simulink library "VariableOrderDifferentialEquationsToolbox"  (R2020a)
settings: Solver=VariableStepAuto  StartTime=0.0  StopTime=10.0  RelTol=1e-3
(part 1 of 3)
settings Model: Creator=dell-wi  LastModifiedBy=Pio
settings DataIOCC: ReturnWorkspaceOutputs=off
settings DebuggingCC: ArithmeticOperatorsInVariantConditions=warning
settings SFSimCC: SimUseLocalCustomCode=off  CustomCodeUndefinedFunction=UseInterfaceOnly
settings RTWCC: RTWUseLocalCustomCode=off

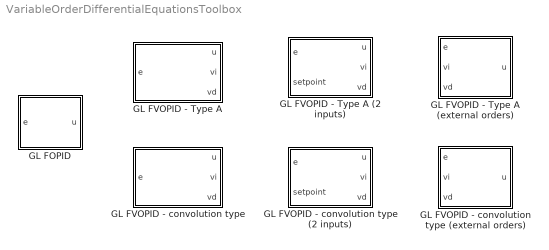
== system VariableOrderDifferentialEquationsToolbox ==
  GL FOPID : Subsystem  mask{kp=1, ki=1, kd=0, sampleTime=1, inputBufferSize=-1, constantIntegralOrder=1, constantDerivativeOrder=1, satEnab=off, satHigh=inf, satLow=-inf}
      mask prompts: kp "Proportional (P)"; ki "Integral (I)"; kd "Derivative (D)"; sampleTime "Sample time"; inputBufferSize "Input buffer size (-1 for automatically calculated)"; constantIntegralOrder "Integral order"; constantDerivativeOrder "Derivative order"; satEnab "Limit output"; satHigh "Upper limit"; satLow "Lower limit"
      mask init:
      | % Initialize block parameters
      | fvopidToolbox.library.utils.initializeBasicModelParameters(sampleTime, inputBufferSize,'fopid');
      settings: CopyFcn=set_param(gcbh, 'LinkStatus', 'none');
      mask Callback satEnab:
      | limitOutputCheckBoxValue = get_param(gcb,'satEnab');
      | if strcmp(limitOutputCheckBoxValue, 'on')
      |    fvopidToolbox.library.utils.setMaskParameterPropertyValue('satHigh', 'MaskEnables', 'on');
      |    fvopidToolbox.library.utils.setMaskParameterPropertyValue('satLow', 'MaskEnables', 'on');
      | else
      |    fvopidToolbox.library.utils.setMaskParameterPropertyValue('satHigh', 'MaskEnables', 'off');
      |    fvopidToolbox.library.utils.setMaskParameterPropertyValue('satLow', 'MaskEnables', 'off');
      | end
      mask DialogControl mainTab Prompt: Main
      mask DialogControl controllerParametersGroupBox Prompt: Controller parameters
      mask DialogControl outputSaturationTab Prompt: Output saturation
      mask DialogControl outputSaturationGroupBox Prompt: Output saturation
  GL FVOPID - Type A : Subsystem  mask{kp=1, ki=1, kd=0, sampleTime=1, inputBufferSize=-1, satEnab=off, satHigh=inf, satLow=-inf, integralOrderTypePopup=Constant order, constantIntegralOrder=1, integralErrorToSetpointRatio=off, integralErrorValuesVector=[0.2, 0.4, 0.6, 0.8], integralOrderValuesVector=[1, 2, 3, 4, 5], timeDependentIntegralOrderExpression=3 * t + 2 * e, derivativeOrderTypePopup=Constant order, constantDerivativeOrder=1, derivativeErrorToSetpointRatio=off, derivativeErrorValuesVector=[0.2, 0.4, 0.6, 0.8], derivativeOrderValuesVector=[1, 2, 3, 4, 5], timeDependentDerivativeOrderExpression=2*t + e}
      mask prompts: kp "Proportional (P)"; ki "Integral (I)"; kd "Derivative (D)"; sampleTime "Sample time"; inputBufferSize "Input buffer size (-1 for automatically calculated)"; satEnab "Limit output"; satHigh "Upper limit"; satLow "Lower limit"; integralOrderTypePopup "Integral order type"; constantIntegralOrder "Integral order"; integralErrorToSetpointRatio "Use error/setpoint ratio"; integralErrorValuesVector "Vector of control error values"; integralOrderValuesVector "Vector of order values"; derivativeOrderTypePopup "Derivative order type"; constantDerivativeOrder "Derivative order"; derivativeErrorToSetpointRatio "Use error/setpoint ratio"; derivativeErrorValuesVector "Vector of control error values"; derivativeOrderValuesVector "Vector of order values"
      mask init:
      | % Initialize block parameters
      | fvopidToolbox.library.utils.initializeBasicModelParameters(sampleTime, inputBufferSize,'fvopidOptimized');
      | integralOrderTypeComboBoxValue = get_param(gcb,'integralOrderTypePopup');
      | derivativeOrderTypeComboBoxValue = get_param(gcb,'derivativeOrderTypePopup');
      | 
      | % Set order function type
      | switch integralOrderTypeComboBoxValue
      |     case 'Constant order'
      |         integralOrderType = 1;
      |     case 'Function of control error'
      |         integralErrorToSetpointRatioValue = get_param(gcb,'integralErrorToSetpointRatio');
      |         if strcmp(integralErrorToSetpointRatioValue, 'on')
      |             integralOrderType = 3;
      |         else
      |             integralOrderType = 2;
      |         end
      |     otherwise
      |         integralOrderExpressionCode = get_param(gcb,'timeDependentIntegralOrderExpression');
      |         newScript = sprintf(['function y = integralTimeDependentMatlabFunction(t, e)\n'...
      |             'y = '  integralOrderExpressionCode ';\nend']);
      |         fvopidToolbox.utils.updateMatlabFunctionBlockScript('integralTimeDependentBlock', newScript,...
      |             [gcb '/integralTimeDependentSubsystem/integralTimeDependentBlock']);
      |         integralOrderType = 4;
      | end
      | 
      | switch derivativeOrderTypeComboBoxValue
      |     case 'Constant order'
      |         derivativeOrderType = 1;
      |     case 'Function of control error'
      |         derivatieErrorToSetpointRatioValue = get_param(gcb,'derivativeErrorToSetpointRatio');
      |         if strcmp(derivatieErrorToSetpointRatioValue, 'on')
      |             derivativeOrderType = 3;
      |         else
      |             derivativeOrderType = 2;
      |         end
      |     otherwise
      |         derivativeOrderExpressionCode = get_param(gcb,'timeDependentDerivativeOrderExpression');
      |         newScript = sprintf(['function y = derivativeTimeDependentMatlabFunction(t, e)\n'...
      |             'y = ' derivativeOrderExpressionCode ';\nend']);
      |         fvopidToolbox.utils.updateMatlabFunctionBlockScript('derivativeTimeDependentBlock', newScript,...
      |             [gcb '/derivativeTimeDependentSubsystem/derivativeTimeDependentBlock']);
      |         derivativeOrderType = 4;
      | end
      | 
      | % Update the input ports
      | setpointInputBlock = find_system(gcb,...
      |     'LookUnderMasks','on',...
      |     'FollowLinks','on','Name','setpointInput');
      | 
      | integralSetpointHolderBlock = find_system(gcb,...
      |     'LookUnderMasks','on',...
      |     'FollowLinks','on','Name','integral_setpoint_placeHolder');
      | 
      | derivativeSetpointHolderBlock = find_system(gcb,...
      |     'LookUnderMasks','on',...
      |     'FollowLinks','on','Name','derivative_setpoint_placeHolder');
      | 
      | if integralOrderType == 3 || derivativeOrderType == 3
      |     if isempty(setpointInputBlock)
      |         add_block('built-in/Inport',[gcb,'/setpointInput']);  
      |     else
      |         h = get_param([gcb '/setpointInput'], 'LineHandles'); 
      |         delete_line(h.Outport(1));
      |     end
      | 
      |     if integralOrderType == 3
      |         if ~isempty(integralSetpointHolderBlock)
      |             h = get_param([gcb '/integral_setpoint_placeHolder'], 'LineHandles'); 
      |             delete_line(h.Outport(1));
      |             delete_block(integralSetpointHolderBlock);
      |         end
      |         add_line(gcb,'setpointInput/1','integralRatioDependentSubsystem/2');
      |     else
      |         if isempty(integralSetpointHolderBlock)
      |             add_block('built-in/Constant',[gcb,'/integral_setpoint_placeHolder']);
      |             set_param([gcb '/integral_setpoint_placeHolder'], 'Value', '0');
      |             add_line(gcb,'integral_setpoint_placeHolder/1','integralRatioDependentSubsystem/2');
      |         end
      |     end
      | 
      |     if derivativeOrderType == 3
      |         if ~isempty(derivativeSetpointHolderBlock)
      |             h = get_param([gcb '/derivative_setpoint_placeHolder'], 'LineHandles'); 
      |             delete_line(h.Outport(1));
      |             delete_block(derivativeSetpointHolderBlock);
      |         end
      |         add_line(gcb,'setpointInput/1','derivativeRatioDependentSubsystem/2');
      |     else
      |         if isempty(derivativeSetpointHolderBlock)
      |             add_block('built-in/Constant',[gcb,'/derivative_setpoint_placeHolder']);
      |             set_param([gcb '/derivative_setpoint_placeHolder'], 'Value', '0');
      |             add_line(gcb,'derivative_setpoint_placeHolder/1','derivativeRatioDependentSubsystem/2');
      |         end
      |     end
      | else
      |     if ~isempty(setpointInputBlock)
      |         h = get_param([gcb '/setpointInput'], 'LineHandles'); 
      |         delete_line(h.Outport(1));
      |         delete_block(setpointInputBlock);
      |     end
      |     
      |     if isempty(integralSetpointHolderBlock)
      |         add_block('built-in/Constant',[gcb,'/integral_setpoint_placeHolder']);
      |         set_param([gcb '/integral_setpoint_placeHolder'], 'Value', '0');
      |         add_line(gcb,'integral_setpoint_placeHolder/1','integralRatioDependentSubsystem/2');
      |     end
      |     
      |     if isempty(derivativeSetpointHolderBlock)
      |         add_block('built-in/Constant',[gcb,'/derivative_setpoint_placeHolder']);
      |         set_param([gcb '/derivative_setpoint_placeHolder'], 'Value', '0');
      |         add_line(gcb,'derivative_setpoint_placeHolder/1','derivativeRatioDependentSubsystem/2');
      |     end
      | end
      settings: CopyFcn=set_param(gcbh, 'LinkStatus', 'none');
      mask Callback satEnab:
      | limitOutputCheckBoxValue = get_param(gcb,'satEnab');
      | if strcmp(limitOutputCheckBoxValue, 'on')
      |    fvopidToolbox.library.utils.setMaskParameterPropertyValue('satHigh', 'MaskEnables', 'on');
      |    fvopidToolbox.library.utils.setMaskParameterPropertyValue('satLow', 'MaskEnables', 'on');
      | else
      |    fvopidToolbox.library.utils.setMaskParameterPropertyValue('satHigh', 'MaskEnables', 'off');
      |    fvopidToolbox.library.utils.setMaskParameterPropertyValue('satLow', 'MaskEnables', 'off');
      | end
      mask TypeOptions integralOrderTypePopup: Constant order | Function of control error | User defined expression
      mask Callback integralOrderTypePopup:
      | selectedComboBoxValue = get_param(gcb,'integralOrderTypePopup');
      | 
      | switch selectedComboBoxValue
      |     case 'Constant order'
      |         fvopidToolbox.library.utils.setMaskElementVisiblePropertyValue('constantIntegralOrderPanel', 'on');
      |         fvopidToolbox.library.utils.setMaskElementVisiblePropertyValue('controlErrorDependentIntegralOrderPanel', 'off');
      |         fvopidToolbox.library.utils.setMaskElementVisiblePropertyValue('timeDependentIntegralOrderPanel', 'off');
      |     case 'Function of control error'
      |         fvopidToolbox.library.utils.setMaskElementVisiblePropertyValue('constantIntegralOrderPanel', 'off');
      |         fvopidToolbox.library.utils.setMaskElementVisiblePropertyValue('controlErrorDependentIntegralOrderPanel', 'on');
      |         fvopidToolbox.library.utils.setMaskElementVisiblePropertyValue('timeDependentIntegralOrderPanel', 'off');
      |     otherwise
      |         fvopidToolbox.library.utils.setMaskElementVisiblePropertyValue('constantIntegralOrderPanel', 'off');
      |         fvopidToolbox.library.utils.setMaskElementVisiblePropertyValue('controlErrorDependentIntegralOrderPanel', 'off');
      |         fvopidToolbox.library.utils.setMaskElementVisiblePropertyValue('timeDependentIntegralOrderPanel', 'on');
      | end
      mask TypeOptions derivativeOrderTypePopup: Constant order | Function of control error | User defined expression
      mask Callback derivativeOrderTypePopup:
      | selectedComboBoxValue = get_param(gcb,'derivativeOrderTypePopup');
      | 
      | switch selectedComboBoxValue
      |     case 'Constant order'
      |         fvopidToolbox.library.utils.setMaskElementVisiblePropertyValue('constantDerivativeOrderPanel', 'on');
      |         fvopidToolbox.library.utils.setMaskElementVisiblePropertyValue('controlErrorDependentDerivativeOrderPanel', 'off');
      |         fvopidToolbox.library.utils.setMaskElementVisiblePropertyValue('timeDependentDerivativeOrderPanel', 'off');
      |     case 'Function of control error'
      |         fvopidToolbox.library.utils.setMaskElementVisiblePropertyValue('constantDerivativeOrderPanel', 'off');
      |         fvopidToolbox.library.utils.setMaskElementVisiblePropertyValue('controlErrorDependentDerivativeOrderPanel', 'on');
      |         fvopidToolbox.library.utils.setMaskElementVisiblePropertyValue('timeDependentDerivativeOrderPanel', 'off');
      |     otherwise
      |         fvopidToolbox.library.utils.setMaskElementVisiblePropertyValue('constantDerivativeOrderPanel', 'off');
      |         fvopidToolbox.library.utils.setMaskElementVisiblePropertyValue('controlErrorDependentDerivativeOrderPanel', 'off');
      |         fvopidToolbox.library.utils.setMaskElementVisiblePropertyValue('timeDependentDerivativeOrderPanel', 'on');
      | end
      mask DialogControl mainTab Prompt: Main
      mask DialogControl controllerParametersGroupBox Prompt: Controller parameters
      mask DialogControl outputSaturationTab Prompt: Output saturation
      mask DialogControl outputSaturationGroupBox Prompt: Output saturation
      mask DialogControl integralOrderTab Prompt: Integral order
      mask DialogControl errorDependentIntegralOrderDescription1 Prompt: Provide a vector of control error values and a vector of order vales. Vector of order values should have one element more than the vector of error. E.g. for if the vector of error values is: [e1, e2, e3] and the vector of orders is [o1, o2, o3, o4], then the orders are generated according to the following rule:
      mask DialogControl errorDependentIntegralOrderDescription2 Prompt: - order = o1 for errors < e1,
      mask DialogControl errorDependentIntegralOrderDescription3 Prompt: - order = o2 for e1 <= error < e2,
      mask DialogControl errorDependentIntegralOrderDescription4 Prompt: - order = o3 for e2 <= error < e3,
      mask DialogControl errorDependentIntegralOrderDescription5 Prompt: - order = o4 for error >= e3.
      mask DialogControl timeDependentIntegralOrderDescription1 Prompt: Insert a short expression which returns value of order as a function of time (t) and/or control error (e), e.g.: '2*t + e' (where 't' is current simulation time and 'e' is current value of the control error).
      mask DialogControl derivativeOrderTab Prompt: Derivative order
      mask DialogControl errorDependentDerivativeOrderDescription1 Prompt: Provide a vector of control error values and a vector of order vales. Vector of order values should have one element more than the vector of error. E.g. for if the vector of order values is: [e1, e2, e3] and the vector of orders is [o1, o2, o3, o4], then the orders are generated according to the following rule:
      mask DialogControl errorDependentDerivativeOrderDescription2 Prompt: - order = o1 for errors > e1,
      mask DialogControl errorDependentDerivativeOrderDescription3 Prompt: - order = o2 for e2 < error <= e1,
      mask DialogControl errorDependentDerivativeOrderDescription4 Prompt: - order = o3 for e3 < error <= e2,
      mask DialogControl errorDependentDerivativeOrderDescription5 Prompt: - order = o4 for error < e3.
      mask DialogControl timeDependentDerivativeOrderDescription1 Prompt: Insert short expression which returns value of order as a function of time (t) and/or control error (e), e.g.: '2*t + e' (where 't' is current simulation time and 'e' is current value of the control error).
  GL FVOPID - Type A (2 inputs) : Subsystem  mask{kp=1, ki=1, kd=0, sampleTime=1, inputBufferSize=-1, satEnab=off, satHigh=inf, satLow=-inf, integralOrderTypePopup=Constant order, constantIntegralOrder=1, integralErrorToSetpointRatio=off, integralErrorValuesVector=[0.2, 0.4, 0.6, 0.8], integralOrderValuesVector=[1, 2, 3, 4, 5], timeDependentIntegralOrderExpression=3 * t + 2 * e, derivativeOrderTypePopup=Constant order, constantDerivativeOrder=1, derivativeErrorToSetpointRatio=off, derivativeErrorValuesVector=[0.2, 0.4, 0.6, 0.8], derivativeOrderValuesVector=[1, 2, 3, 4, 5], timeDependentDerivativeOrderExpression=2*t + e}
      mask prompts: kp "Proportional (P)"; ki "Integral (I)"; kd "Derivative (D)"; sampleTime "Sample time"; inputBufferSize "Input buffer size (-1 for automatically calculated)"; satEnab "Limit output"; satHigh "Upper limit"; satLow "Lower limit"; integralOrderTypePopup "Integral order type"; constantIntegralOrder "Integral order"; integralErrorToSetpointRatio "Use error/setpoint ratio"; integralErrorValuesVector "Vector of control error values"; integralOrderValuesVector "Vector of order values"; derivativeOrderTypePopup "Derivative order type"; constantDerivativeOrder "Derivative order"; derivativeErrorToSetpointRatio "Use error/setpoint ratio"; derivativeErrorValuesVector "Vector of control error values"; derivativeOrderValuesVector "Vector of order values"
      mask init:
      | % Initialize block parameters
      | fvopidToolbox.library.utils.initializeBasicModelParameters(sampleTime, inputBufferSize,'fvopidOptimized');
      | integralOrderTypeComboBoxValue = get_param(gcb,'integralOrderTypePopup');
      | derivativeOrderTypeComboBoxValue = get_param(gcb,'derivativeOrderTypePopup');
      | 
      | % Set order function type
      | switch integralOrderTypeComboBoxValue
      |     case 'Constant order'
      |         integralOrderType = 1;
      |     case 'Function of control error'
      |         integralErrorToSetpointRatioValue = get_param(gcb,'integralErrorToSetpointRatio');
      |         if strcmp(integralErrorToSetpointRatioValue, 'on')
      |             integralOrderType = 3;
      |         else
      |             integralOrderType = 2;
      |         end
      |     otherwise
      |         integralOrderExpressionCode = get_param(gcb,'timeDependentIntegralOrderExpression');
      |         newScript = sprintf(['function y = integralTimeDependentMatlabFunction(t, e)\n'...
      |             'y = '  integralOrderExpressionCode ';\nend']);
      |         fvopidToolbox.utils.updateMatlabFunctionBlockScript('integralTimeDependentBlock', newScript,...
      |             [gcb '/integralTimeDependentSubsystem/integralTimeDependentBlock']);
      |         integralOrderType = 4;
      | end
      | 
      | switch derivativeOrderTypeComboBoxValue
      |     case 'Constant order'
      |         derivativeOrderType = 1;
      |     case 'Function of control error'
      |         derivatieErrorToSetpointRatioValue = get_param(gcb,'derivativeErrorToSetpointRatio');
      |         if strcmp(derivatieErrorToSetpointRatioValue, 'on')
      |             derivativeOrderType = 3;
      |         else
      |             derivativeOrderType = 2;
      |         end
      |     otherwise
      |         derivativeOrderExpressionCode = get_param(gcb,'timeDependentDerivativeOrderExpression');
      |         newScript = sprintf(['function y = derivativeTimeDependentMatlabFunction(t, e)\n'...
      |             'y = ' derivativeOrderExpressionCode ';\nend']);
      |         fvopidToolbox.utils.updateMatlabFunctionBlockScript('derivativeTimeDependentBlock', newScript,...
      |             [gcb '/derivativeTimeDependentSubsystem/derivativeTimeDependentBlock']);
      |         derivativeOrderType = 4;
      | end
      | 
      | % Update the input ports
      | setpointInputBlock = find_system(gcb,...
      |     'LookUnderMasks','on',...
      |     'FollowLinks','on','Name','setpointInput');
      | if integralOrderType == 3 || derivativeOrderType == 3
      |     if isempty(setpointInputBlock)
      |         add_block('built-in/Inport',[gcb,'/setpointInput']);  
      |     else
      |         h = get_param([gcb '/setpointInput'], 'LineHandles'); 
      |         delete_line(h.Outport(1));
      |     end
      | 
      |     if integralOrderType == 3
      |         add_line(gcb,'setpointInput/1','integralRatioDependentSubsystem/2');
      |     end
      | 
      |     if derivativeOrderType == 3
      |         add_line(gcb,'setpointInput/1','derivativeRatioDependentSubsystem/2');
      |     end
      | else
      |     if ~isempty(setpointInputBlock)
      |         h = get_param([gcb '/setpointInput'], 'LineHandles'); 
      |         delete_line(h.Outport(1));
      |         delete_block(setpointInputBlock);
      |     end
      | end
      settings: CopyFcn=set_param(gcbh, 'LinkStatus', 'none');
      mask Callback satEnab:
      | limitOutputCheckBoxValue = get_param(gcb,'satEnab');
      | if strcmp(limitOutputCheckBoxValue, 'on')
      |    fvopidToolbox.library.utils.setMaskParameterPropertyValue('satHigh', 'MaskEnables', 'on');
      |    fvopidToolbox.library.utils.setMaskParameterPropertyValue('satLow', 'MaskEnables', 'on');
      | else
      |    fvopidToolbox.library.utils.setMaskParameterPropertyValue('satHigh', 'MaskEnables', 'off');
      |    fvopidToolbox.library.utils.setMaskParameterPropertyValue('satLow', 'MaskEnables', 'off');
      | end
      mask TypeOptions integralOrderTypePopup: Constant order | Function of control error | User defined expression
      mask Callback integralOrderTypePopup:
      | selectedComboBoxValue = get_param(gcb,'integralOrderTypePopup');
      | 
      | switch selectedComboBoxValue
      |     case 'Constant order'
      |         fvopidToolbox.library.utils.setMaskElementVisiblePropertyValue('constantIntegralOrderPanel', 'on');
      |         fvopidToolbox.library.utils.setMaskElementVisiblePropertyValue('controlErrorDependentIntegralOrderPanel', 'off');
      |         fvopidToolbox.library.utils.setMaskElementVisiblePropertyValue('timeDependentIntegralOrderPanel', 'off');
      |     case 'Function of control error'
      |         fvopidToolbox.library.utils.setMaskElementVisiblePropertyValue('constantIntegralOrderPanel', 'off');
      |         fvopidToolbox.library.utils.setMaskElementVisiblePropertyValue('controlErrorDependentIntegralOrderPanel', 'on');
      |         fvopidToolbox.library.utils.setMaskElementVisiblePropertyValue('timeDependentIntegralOrderPanel', 'off');
      |     otherwise
      |         fvopidToolbox.library.utils.setMaskElementVisiblePropertyValue('constantIntegralOrderPanel', 'off');
      |         fvopidToolbox.library.utils.setMaskElementVisiblePropertyValue('controlErrorDependentIntegralOrderPanel', 'off');
      |         fvopidToolbox.library.utils.setMaskElementVisiblePropertyValue('timeDependentIntegralOrderPanel', 'on');
      | end
      mask TypeOptions derivativeOrderTypePopup: Constant order | Function of control error | User defined expression
      mask Callback derivativeOrderTypePopup:
      | selectedComboBoxValue = get_param(gcb,'derivativeOrderTypePopup');
      | 
      | switch selectedComboBoxValue
      |     case 'Constant order'
      |         fvopidToolbox.library.utils.setMaskElementVisiblePropertyValue('constantDerivativeOrderPanel', 'on');
      |         fvopidToolbox.library.utils.setMaskElementVisiblePropertyValue('controlErrorDependentDerivativeOrderPanel', 'off');
      |         fvopidToolbox.library.utils.setMaskElementVisiblePropertyValue('timeDependentDerivativeOrderPanel', 'off');
      |     case 'Function of control error'
      |         fvopidToolbox.library.utils.setMaskElementVisiblePropertyValue('constantDerivativeOrderPanel', 'off');
      |         fvopidToolbox.library.utils.setMaskElementVisiblePropertyValue('controlErrorDependentDerivativeOrderPanel', 'on');
      |         fvopidToolbox.library.utils.setMaskElementVisiblePropertyValue('timeDependentDerivativeOrderPanel', 'off');
      |     otherwise
      |         fvopidToolbox.library.utils.setMaskElementVisiblePropertyValue('constantDerivativeOrderPanel', 'off');
      |         fvopidToolbox.library.utils.setMaskElementVisiblePropertyValue('controlErrorDependentDerivativeOrderPanel', 'off');
      |         fvopidToolbox.library.utils.setMaskElementVisiblePropertyValue('timeDependentDerivativeOrderPanel', 'on');
      | end
      mask DialogControl mainTab Prompt: Main
      mask DialogControl controllerParametersGroupBox Prompt: Controller parameters
      mask DialogControl outputSaturationTab Prompt: Output saturation
      mask DialogControl outputSaturationGroupBox Prompt: Output saturation
      mask DialogControl integralOrderTab Prompt: Integral order
      mask DialogControl errorDependentIntegralOrderDescription1 Prompt: Provide a vector of control error values and a vector of order vales. Vector of order values should have one element more than the vector of error. E.g. for if the vector of order values is: [e1, e2, e3] and the vector of orders is [o1, o2, o3, o4], then the orders are generated according to the following rule:
      mask DialogControl errorDependentIntegralOrderDescription2 Prompt: - order = o1 for errors > e1,
      mask DialogControl errorDependentIntegralOrderDescription3 Prompt: - order = o2 for e2 < error <= e1,
      mask DialogControl errorDependentIntegralOrderDescription4 Prompt: - order = o3 for e3 < error <= e2,
      mask DialogControl errorDependentIntegralOrderDescription5 Prompt: - order = o4 for error < e3.
      mask DialogControl timeDependentIntegralOrderDescription1 Prompt: Insert short expression which returns value of order as a function of time (t) and/or control error (e), e.g.: '2*t + e' (where 't' is current simulation time and 'e' is current value of the control error).
      mask DialogControl derivativeOrderTab Prompt: Derivative order
      mask DialogControl errorDependentDerivativeOrderDescription1 Prompt: Provide a vector of control error values and a vector of order vales. Vector of order values should have one element more than the vector of error. E.g. for if the vector of order values is: [e1, e2, e3] and the vector of orders is [o1, o2, o3, o4], then the orders are generated according to the following rule:
      mask DialogControl errorDependentDerivativeOrderDescription2 Prompt: - order = o1 for errors > e1,
      mask DialogControl errorDependentDerivativeOrderDescription3 Prompt: - order = o2 for e2 < error <= e1,
      mask DialogControl errorDependentDerivativeOrderDescription4 Prompt: - order = o3 for e3 < error <= e2,
      mask DialogControl errorDependentDerivativeOrderDescription5 Prompt: - order = o4 for error < e3.
      mask DialogControl timeDependentDerivativeOrderDescription1 Prompt: Insert short expression which returns value of order as a function of time (t) and/or control error (e), e.g.: '2*t + e' (where 't' is current simulation time and 'e' is current value of the control error).
  GL FVOPID - Type A (external orders) : Subsystem  mask{kp=1, ki=1, kd=0, sampleTime=1, inputBufferSize=-1, satEnab=off, satHigh=inf, satLow=-inf}
      mask prompts: kp "Proportional (P)"; ki "Integral (I)"; kd "Derivative (D)"; sampleTime "Sample time"; inputBufferSize "Input buffer size (-1 for automatically calculated)"; satEnab "Limit output"; satHigh "Upper limit"; satLow "Lower limit"
      mask init:
      | % Initialize block parameters
      | fvopidToolbox.library.utils.initializeBasicModelParameters(sampleTime, inputBufferSize,'fvopidOptimized');
      settings: CopyFcn=set_param(gcbh, 'LinkStatus', 'none');
      mask Callback satEnab:
      | limitOutputCheckBoxValue = get_param(gcb,'satEnab');
      | if strcmp(limitOutputCheckBoxValue, 'on')
      |    fvopidToolbox.library.utils.setMaskParameterPropertyValue('satHigh', 'MaskEnables', 'on');
      |    fvopidToolbox.library.utils.setMaskParameterPropertyValue('satLow', 'MaskEnables', 'on');
      | else
      |    fvopidToolbox.library.utils.setMaskParameterPropertyValue('satHigh', 'MaskEnables', 'off');
      |    fvopidToolbox.library.utils.setMaskParameterPropertyValue('satLow', 'MaskEnables', 'off');
      | end
      mask DialogControl mainTab Prompt: Main
      mask DialogControl controllerParametersGroupBox Prompt: Controller parameters
      mask DialogControl outputSaturationTab Prompt: Output saturation
      mask DialogControl outputSaturationGroupBox Prompt: Output saturation
  GL FVOPID - convolution type : Subsystem  mask{kp=1, ki=1, kd=0, sampleTime=1, inputBufferSize=-1, satEnab=off, satHigh=inf, satLow=-inf, integralOrderTypePopup=Constant order, constantIntegralOrder=1, integralErrorToSetpointRatio=off, integralErrorValuesVector=[0.2, 0.4, 0.6, 0.8], integralOrderValuesVector=[1, 2, 3, 4, 5], timeDependentIntegralOrderExpression=3 * t + 2 * e, derivativeOrderTypePopup=Constant order, constantDerivativeOrder=1, derivativeErrorToSetpointRatio=off, derivativeErrorValuesVector=[0.2, 0.4, 0.6, 0.8], derivativeOrderValuesVector=[1, 2, 3, 4, 5], timeDependentDerivativeOrderExpression=2*t + e}
      mask prompts: kp "Proportional (P)"; ki "Integral (I)"; kd "Derivative (D)"; sampleTime "Sample time"; inputBufferSize "Input buffer size (-1 for automatically calculated)"; satEnab "Limit output"; satHigh "Upper limit"; satLow "Lower limit"; integralOrderTypePopup "Integral order type"; constantIntegralOrder "Integral order"; integralErrorToSetpointRatio "Use error/setpoint ratio"; integralErrorValuesVector "Vector of control error values"; integralOrderValuesVector "Vector of order values"; derivativeOrderTypePopup "Derivative order type"; constantDerivativeOrder "Derivative order"; derivativeErrorToSetpointRatio "Use error/setpoint ratio"; derivativeErrorValuesVector "Vector of control error values"; derivativeOrderValuesVector "Vector of order values"
      mask init:
      | % Initialize block parameters
      | fvopidToolbox.library.utils.initializeBasicModelParameters(sampleTime, inputBufferSize,'fvopidConv');
      | integralOrderTypeComboBoxValue = get_param(gcb,'integralOrderTypePopup');
      | derivativeOrderTypeComboBoxValue = get_param(gcb,'derivativeOrderTypePopup');
      | 
      | % Set order function type
      | switch integralOrderTypeComboBoxValue
      |     case 'Constant order'
      |         integralOrderType = 1;
      |     case 'Function of control error'
      |         integralErrorToSetpointRatioValue = get_param(gcb,'integralErrorToSetpointRatio');
      |         if strcmp(integralErrorToSetpointRatioValue, 'on')
      |             integralOrderType = 3;
      |         else
      |             integralOrderType = 2;
      |         end
      |     otherwise
      |         integralOrderExpressionCode = get_param(gcb,'timeDependentIntegralOrderExpression');
      |         newScript = sprintf(['function y = integralTimeDependentMatlabFunction(t, e)\n'...
      |             'y = '  integralOrderExpressionCode ';\nend']);
      |         fvopidToolbox.utils.updateMatlabFunctionBlockScript('integralTimeDependentBlock', newScript,...
      |             [gcb '/integralTimeDependentSubsystem/integralTimeDependentBlock']);
      |         integralOrderType = 4;
      | end
      | 
      | switch derivativeOrderTypeComboBoxValue
      |     case 'Constant order'
      |         derivativeOrderType = 1;
      |     case 'Function of control error'
      |         derivatieErrorToSetpointRatioValue = get_param(gcb,'derivativeErrorToSetpointRatio');
      |         if strcmp(derivatieErrorToSetpointRatioValue, 'on')
      |             derivativeOrderType = 3;
      |         else
      |             derivativeOrderType = 2;
      |         end
      |     otherwise
      |         derivativeOrderExpressionCode = get_param(gcb,'timeDependentDerivativeOrderExpression');
      |         newScript = sprintf(['function y = derivativeTimeDependentMatlabFunction(t, e)\n'...
      |             'y = ' derivativeOrderExpressionCode ';\nend']);
      |         fvopidToolbox.utils.updateMatlabFunctionBlockScript('derivativeTimeDependentBlock', newScript,...
      |             [gcb '/derivativeTimeDependentSubsystem/derivativeTimeDependentBlock']);
      |         derivativeOrderType = 4;
      | end
      | 
      | % Update the input ports
      | setpointInputBlock = find_system(gcb,...
      |     'LookUnderMasks','on',...
      |     'FollowLinks','on','Name','setpointInput');
      | 
      | integralSetpointHolderBlock = find_system(gcb,...
      |     'LookUnderMasks','on',...
      |     'FollowLinks','on','Name','integral_setpoint_placeHolder');
      | 
      | derivativeSetpointHolderBlock = find_system(gcb,...
      |     'LookUnderMasks','on',...
      |     'FollowLinks','on','Name','derivative_setpoint_placeHolder');
      | 
      | if integralOrderType == 3 || derivativeOrderType == 3
      |     if isempty(setpointInputBlock)
      |         add_block('built-in/Inport',[gcb,'/setpointInput']);  
      |     else
      |         h = get_param([gcb '/setpointInput'], 'LineHandles'); 
      |         delete_line(h.Outport(1));
      |     end
      | 
      |     if integralOrderType == 3
      |         if ~isempty(integralSetpointHolderBlock)
      |             h = get_param([gcb '/integral_setpoint_placeHolder'], 'LineHandles'); 
      |             delete_line(h.Outport(1));
      |             delete_block(integralSetpointHolderBlock);
      |         end
      |         add_line(gcb,'setpointInput/1','integralRatioDependentSubsystem/2');
      |     else
      |         if isempty(integralSetpointHolderBlock)
      |             add_block('built-in/Constant',[gcb,'/integral_setpoint_placeHolder']);
      |             set_param([gcb '/integral_setpoint_placeHolder'], 'Value', '0');
      |             add_line(gcb,'integral_setpoint_placeHolder/1','integralRatioDependentSubsystem/2');
      |         end
      |     end
      | 
      |     if derivativeOrderType == 3
      |         if ~isempty(derivativeSetpointHolderBlock)
      |             h = get_param([gcb '/derivative_setpoint_placeHolder'], 'LineHandles'); 
      |             delete_line(h.Outport(1));
      |             delete_block(derivativeSetpointHolderBlock);
      |         end
      |         add_line(gcb,'setpointInput/1','derivativeRatioDependentSubsystem/2');
      |     else
      |         if isempty(derivativeSetpointHolderBlock)
      |             add_block('built-in/Constant',[gcb,'/derivative_setpoint_placeHolder']);
      |             set_param([gcb '/derivative_setpoint_placeHolder'], 'Value', '0');
      |             add_line(gcb,'derivative_setpoint_placeHolder/1','derivativeRatioDependentSubsystem/2');
      |         end
      |     end
      | else
      |     if ~isempty(setpointInputBlock)
      |         h = get_param([gcb '/setpointInput'], 'LineHandles'); 
      |         delete_line(h.Outport(1));
      |         delete_block(setpointInputBlock);
      |     end
      |     
      |     if isempty(integralSetpointHolderBlock)
      |         add_block('built-in/Constant',[gcb,'/integral_setpoint_placeHolder']);
      |         set_param([gcb '/integral_setpoint_placeHolder'], 'Value', '0');
      |         add_line(gcb,'integral_setpoint_placeHolder/1','integralRatioDependentSubsystem/2');
      |     end
      |     
      |     if isempty(derivativeSetpointHolderBlock)
      |         add_block('built-in/Constant',[gcb,'/derivative_setpoint_placeHolder']);
      |         set_param([gcb '/derivative_setpoint_placeHolder'], 'Value', '0');
      |         add_line(gcb,'derivative_setpoint_placeHolder/1','derivativeRatioDependentSubsystem/2');
      |     end
      | end
      settings: CopyFcn=set_param(gcbh, 'LinkStatus', 'none');
      mask Callback satEnab:
      | limitOutputCheckBoxValue = get_param(gcb,'satEnab');
      | if strcmp(limitOutputCheckBoxValue, 'on')
      |    fvopidToolbox.library.utils.setMaskParameterPropertyValue('satHigh', 'MaskEnables', 'on');
      |    fvopidToolbox.library.utils.setMaskParameterPropertyValue('satLow', 'MaskEnables', 'on');
      | else
      |    fvopidToolbox.library.utils.setMaskParameterPropertyValue('satHigh', 'MaskEnables', 'off');
      |    fvopidToolbox.library.utils.setMaskParameterPropertyValue('satLow', 'MaskEnables', 'off');
      | end
      mask TypeOptions integralOrderTypePopup: Constant order | Function of control error | User defined expression
      mask Callback integralOrderTypePopup:
      | selectedComboBoxValue = get_param(gcb,'integralOrderTypePopup');
      | 
      | switch selectedComboBoxValue
      |     case 'Constant order'
      |         fvopidToolbox.library.utils.setMaskElementVisiblePropertyValue('constantIntegralOrderPanel', 'on');
      |         fvopidToolbox.library.utils.setMaskElementVisiblePropertyValue('controlErrorDependentIntegralOrderPanel', 'off');
      |         fvopidToolbox.library.utils.setMaskElementVisiblePropertyValue('timeDependentIntegralOrderPanel', 'off');
      |     case 'Function of control error'
      |         fvopidToolbox.library.utils.setMaskElementVisiblePropertyValue('constantIntegralOrderPanel', 'off');
      |         fvopidToolbox.library.utils.setMaskElementVisiblePropertyValue('controlErrorDependentIntegralOrderPanel', 'on');
      |         fvopidToolbox.library.utils.setMaskElementVisiblePropertyValue('timeDependentIntegralOrderPanel', 'off');
      |     otherwise
      |         fvopidToolbox.library.utils.setMaskElementVisiblePropertyValue('constantIntegralOrderPanel', 'off');
      |         fvopidToolbox.library.utils.setMaskElementVisiblePropertyValue('controlErrorDependentIntegralOrderPanel', 'off');
      |         fvopidToolbox.library.utils.setMaskElementVisiblePropertyValue('timeDependentIntegralOrderPanel', 'on');
      | end
      mask TypeOptions derivativeOrderTypePopup: Constant order | Function of control error | User defined expression
      mask Callback derivativeOrderTypePopup:
      | selectedComboBoxValue = get_param(gcb,'derivativeOrderTypePopup');
      | 
      | switch selectedComboBoxValue
      |     case 'Constant order'
      |         fvopidToolbox.library.utils.setMaskElementVisiblePropertyValue('constantDerivativeOrderPanel', 'on');
      |         fvopidToolbox.library.utils.setMaskElementVisiblePropertyValue('controlErrorDependentDerivativeOrderPanel', 'off');
      |         fvopidToolbox.library.utils.setMaskElementVisiblePropertyValue('timeDependentDerivativeOrderPanel', 'off');
      |     case 'Function of control error'
      |         fvopidToolbox.library.utils.setMaskElementVisiblePropertyValue('constantDerivativeOrderPanel', 'off');
      |         fvopidToolbox.library.utils.setMaskElementVisiblePropertyValue('controlErrorDependentDerivativeOrderPanel', 'on');
      |         fvopidToolbox.library.utils.setMaskElementVisiblePropertyValue('timeDependentDerivativeOrderPanel', 'off');
      |     otherwise
      |         fvopidToolbox.library.utils.setMaskElementVisiblePropertyValue('constantDerivativeOrderPanel', 'off');
      |         fvopidToolbox.library.utils.setMaskElementVisiblePropertyValue('controlErrorDependentDerivativeOrderPanel', 'off');
      |         fvopidToolbox.library.utils.setMaskElementVisiblePropertyValue('timeDependentDerivativeOrderPanel', 'on');
      | end
      mask DialogControl mainTab Prompt: Main
      mask DialogControl controllerParametersGroupBox Prompt: Controller parameters
      mask DialogControl outputSaturationTab Prompt: Output saturation
      mask DialogControl outputSaturationGroupBox Prompt: Output saturation
      mask DialogControl integralOrderTab Prompt: Integral order
      mask DialogControl errorDependentIntegralOrderDescription1 Prompt: Provide a vector of control error values and a vector of order vales. Vector of order values should have one element more than the vector of error. E.g. for if the vector of order values is: [e1, e2, e3] and the vector of orders is [o1, o2, o3, o4], then the orders are generated according to the following rule:
      mask DialogControl errorDependentIntegralOrderDescription2 Prompt: - order = o1 for errors > e1,
      mask DialogControl errorDependentIntegralOrderDescription3 Prompt: - order = o2 for e2 < error <= e1,
      mask DialogControl errorDependentIntegralOrderDescription4 Prompt: - order = o3 for e3 < error <= e2,
      mask DialogControl errorDependentIntegralOrderDescription5 Prompt: - order = o4 for error < e3.
      mask DialogControl timeDependentIntegralOrderDescription1 Prompt: Insert short expression which returns value of order as a function of time (t) and/or control error (e), e.g.: '2*t + e' (where 't' is current simulation time and 'e' is current value of the control error).
      mask DialogControl derivativeOrderTab Prompt: Derivative order
      mask DialogControl errorDependentDerivativeOrderDescription1 Prompt: Provide a vector of control error values and a vector of order vales. Vector of order values should have one element more than the vector of error. E.g. for if the vector of order values is: [e1, e2, e3] and the vector of orders is [o1, o2, o3, o4], then the orders are generated according to the following rule:
      mask DialogControl errorDependentDerivativeOrderDescription2 Prompt: - order = o1 for errors > e1,
      mask DialogControl errorDependentDerivativeOrderDescription3 Prompt: - order = o2 for e2 < error <= e1,
      mask DialogControl errorDependentDerivativeOrderDescription4 Prompt: - order = o3 for e3 < error <= e2,
      mask DialogControl errorDependentDerivativeOrderDescription5 Prompt: - order = o4 for error < e3.
      mask DialogControl timeDependentDerivativeOrderDescription1 Prompt: Insert short expression which returns value of order as a function of time (t) and/or control error (e), e.g.: '2*t + e' (where 't' is current simulation time and 'e' is current value of the control error).
  GL FVOPID - convolution type (2 inputs) : Subsystem  mask{kp=1, ki=1, kd=0, sampleTime=1, inputBufferSize=-1, satEnab=off, satHigh=inf, satLow=-inf, integralOrderTypePopup=Constant order, constantIntegralOrder=1, integralErrorToSetpointRatio=off, integralErrorValuesVector=[0.2, 0.4, 0.6, 0.8], integralOrderValuesVector=[1, 2, 3, 4, 5], timeDependentIntegralOrderExpression=3 * t + 2 * e, derivativeOrderTypePopup=Constant order, constantDerivativeOrder=1, derivativeErrorToSetpointRatio=off, derivativeErrorValuesVector=[0.2, 0.4, 0.6, 0.8], derivativeOrderValuesVector=[1, 2, 3, 4, 5], timeDependentDerivativeOrderExpression=2*t + e}
      mask prompts: kp "Proportional (P)"; ki "Integral (I)"; kd "Derivative (D)"; sampleTime "Sample time"; inputBufferSize "Input buffer size (-1 for automatically calculated)"; satEnab "Limit output"; satHigh "Upper limit"; satLow "Lower limit"; integralOrderTypePopup "Integral order type"; constantIntegralOrder "Integral order"; integralErrorToSetpointRatio "Use error/setpoint ratio"; integralErrorValuesVector "Vector of control error values"; integralOrderValuesVector "Vector of order values"; derivativeOrderTypePopup "Derivative order type"; constantDerivativeOrder "Derivative order"; derivativeErrorToSetpointRatio "Use error/setpoint ratio"; derivativeErrorValuesVector "Vector of control error values"; derivativeOrderValuesVector "Vector of order values"
      mask init:
      | % Initialize block parameters
      | fvopidToolbox.library.utils.initializeBasicModelParameters(sampleTime, inputBufferSize,'fvopidConv');
      | integralOrderTypeComboBoxValue = get_param(gcb,'integralOrderTypePopup');
      | derivativeOrderTypeComboBoxValue = get_param(gcb,'derivativeOrderTypePopup');
      | 
      | % Set order function type
      | switch integralOrderTypeComboBoxValue
      |     case 'Constant order'
      |         integralOrderType = 1;
      |     case 'Control error function'
      |         integralErrorToSetpointRatioValue = get_param(gcb,'integralErrorToSetpointRatio');
      |         if strcmp(integralErrorToSetpointRatioValue, 'on')
      |             integralOrderType = 3;
      |         else
      |             integralOrderType = 2;
      |         end
      |     otherwise
      |         integralOrderExpressionCode = get_param(gcb,'timeDependentIntegralOrderExpression');
      |         newScript = sprintf(['function y = integralTimeDependentMatlabFunction(t, e)\n'...
      |             'y = '  integralOrderExpressionCode ';\nend']);
      |         fvopidToolbox.utils.updateMatlabFunctionBlockScript('integralTimeDependentBlock', newScript,...
      |             [gcb '/integralTimeDependentSubsystem/integralTimeDependentBlock']);
      |         integralOrderType = 4;
      | end
      | 
      | switch derivativeOrderTypeComboBoxValue
      |     case 'Constant order'
      |         derivativeOrderType = 1;
      |     case 'Control error function'
      |         derivatieErrorToSetpointRatioValue = get_param(gcb,'derivativeErrorToSetpointRatio');
      |         if strcmp(derivatieErrorToSetpointRatioValue, 'on')
      |             derivativeOrderType = 3;
      |         else
      |             derivativeOrderType = 2;
      |         end
      |     otherwise
      |         derivativeOrderExpressionCode = get_param(gcb,'timeDependentDerivativeOrderExpression');
      |         newScript = sprintf(['function y = derivativeTimeDependentMatlabFunction(t, e)\n'...
      |             'y = ' derivativeOrderExpressionCode ';\nend']);
      |         fvopidToolbox.utils.updateMatlabFunctionBlockScript('derivativeTimeDependentBlock', newScript,...
      |             [gcb '/derivativeTimeDependentSubsystem/derivativeTimeDependentBlock']);
      |         derivativeOrderType = 4;
      | end
      | 
      | % Update the input ports
      | setpointInputBlock = find_system(gcb,...
      |     'LookUnderMasks','on',...
      |     'FollowLinks','on','Name','setpointInput');
      | if integralOrderType == 3 || derivativeOrderType == 3
      |     if isempty(setpointInputBlock)
      |         add_block('built-in/Inport',[gcb,'/setpointInput']);  
      |     else
      |         h = get_param([gcb '/setpointInput'], 'LineHandles'); 
      |         delete_line(h.Outport(1));
      |     end
      | 
      |     if integralOrderType == 3
      |         add_line(gcb,'setpointInput/1','integralRatioDependentSubsystem/2');
      |     end
      | 
      |     if derivativeOrderType == 3
      |         add_line(gcb,'setpointInput/1','derivativeRatioDependentSubsystem/2');
      |     end
      | else
      |     if ~isempty(setpointInputBlock)
      |         h = get_param([gcb '/setpointInput'], 'LineHandles'); 
      |         delete_line(h.Outport(1));
      |         delete_block(setpointInputBlock);
      |     end
      | end
      settings: CopyFcn=set_param(gcbh, 'LinkStatus', 'none');
      mask Callback satEnab:
      | limitOutputCheckBoxValue = get_param(gcb,'satEnab');
      | if strcmp(limitOutputCheckBoxValue, 'on')
      |    fvopidToolbox.library.utils.setMaskParameterPropertyValue('satHigh', 'MaskEnables', 'on');
      |    fvopidToolbox.library.utils.setMaskParameterPropertyValue('satLow', 'MaskEnables', 'on');
      | else
      |    fvopidToolbox.library.utils.setMaskParameterPropertyValue('satHigh', 'MaskEnables', 'off');
      |    fvopidToolbox.library.utils.setMaskParameterPropertyValue('satLow', 'MaskEnables', 'off');
      | end
      mask TypeOptions integralOrderTypePopup: Constant order | Function of control error | User defined expression
      mask Callback integralOrderTypePopup:
      | selectedComboBoxValue = get_param(gcb,'integralOrderTypePopup');
      | 
      | switch selectedComboBoxValue
      |     case 'Constant order'
      |         fvopidToolbox.library.utils.setMaskElementVisiblePropertyValue('constantIntegralOrderPanel', 'on');
      |         fvopidToolbox.library.utils.setMaskElementVisiblePropertyValue('controlErrorDependentIntegralOrderPanel', 'off');
      |         fvopidToolbox.library.utils.setMaskElementVisiblePropertyValue('timeDependentIntegralOrderPanel', 'off');
      |     case 'Function of control error'
      |         fvopidToolbox.library.utils.setMaskElementVisiblePropertyValue('constantIntegralOrderPanel', 'off');
      |         fvopidToolbox.library.utils.setMaskElementVisiblePropertyValue('controlErrorDependentIntegralOrderPanel', 'on');
      |         fvopidToolbox.library.utils.setMaskElementVisiblePropertyValue('timeDependentIntegralOrderPanel', 'off');
      |     otherwise
      |         fvopidToolbox.library.utils.setMaskElementVisiblePropertyValue('constantIntegralOrderPanel', 'off');
      |         fvopidToolbox.library.utils.setMaskElementVisiblePropertyValue('controlErrorDependentIntegralOrderPanel', 'off');
      |         fvopidToolbox.library.utils.setMaskElementVisiblePropertyValue('timeDependentIntegralOrderPanel', 'on');
      | end
      mask TypeOptions derivativeOrderTypePopup: Constant order | Function of control error | User defined expression
      mask Callback derivativeOrderTypePopup:
      | selectedComboBoxValue = get_param(gcb,'derivativeOrderTypePopup');
      | 
      | switch selectedComboBoxValue
      |     case 'Constant order'
      |         fvopidToolbox.library.utils.setMaskElementVisiblePropertyValue('constantDerivativeOrderPanel', 'on');
      |         fvopidToolbox.library.utils.setMaskElementVisiblePropertyValue('controlErrorDependentDerivativeOrderPanel', 'off');
      |         fvopidToolbox.library.utils.setMaskElementVisiblePropertyValue('timeDependentDerivativeOrderPanel', 'off');
      |     case 'Function of control error'
      |         fvopidToolbox.library.utils.setMaskElementVisiblePropertyValue('constantDerivativeOrderPanel', 'off');
      |         fvopidToolbox.library.utils.setMaskElementVisiblePropertyValue('controlErrorDependentDerivativeOrderPanel', 'on');
      |         fvopidToolbox.library.utils.setMaskElementVisiblePropertyValue('timeDependentDerivativeOrderPanel', 'off');
      |     otherwise
      |         fvopidToolbox.library.utils.setMaskElementVisiblePropertyValue('constantDerivativeOrderPanel', 'off');
      |         fvopidToolbox.library.utils.setMaskElementVisiblePropertyValue('controlErrorDependentDerivativeOrderPanel', 'off');
      |         fvopidToolbox.library.utils.setMaskElementVisiblePropertyValue('timeDependentDerivativeOrderPanel', 'on');
      | end
      mask DialogControl mainTab Prompt: Main
      mask DialogControl controllerParametersGroupBox Prompt: Controller parameters
      mask DialogControl outputSaturationTab Prompt: Output saturation
      mask DialogControl outputSaturationGroupBox Prompt: Output saturation
      mask DialogControl integralOrderTab Prompt: Integral order
      mask DialogControl errorDependentIntegralOrderDescription1 Prompt: Provide a vector of control error values and a vector of order vales. Vector of order values should have one element more than the vector of error. E.g. for if the vector of order values is: [e1, e2, e3] and the vector of orders is [o1, o2, o3, o4], then the orders are generated according to the following rule:
      mask DialogControl errorDependentIntegralOrderDescription2 Prompt: - order = o1 for errors > e1,
      mask DialogControl errorDependentIntegralOrderDescription3 Prompt: - order = o2 for e2 < error <= e1,
      mask DialogControl errorDependentIntegralOrderDescription4 Prompt: - order = o3 for e3 < error <= e2,
      mask DialogControl errorDependentIntegralOrderDescription5 Prompt: - order = o4 for error < e3.
      mask DialogControl timeDependentIntegralOrderDescription1 Prompt: Insert short expression which returns value of order as a function of time (t) and/or control error (e), e.g.: '2*t + e' (where 't' is current simulation time and 'e' is current value of the control error).
      mask DialogControl derivativeOrderTab Prompt: Derivative order
      mask DialogControl errorDependentDerivativeOrderDescription1 Prompt: Provide a vector of control error values and a vector of order vales. Vector of order values should have one element more than the vector of error. E.g. for if the vector of order values is: [e1, e2, e3] and the vector of orders is [o1, o2, o3, o4], then the orders are generated according to the following rule:
      mask DialogControl errorDependentDerivativeOrderDescription2 Prompt: - order = o1 for errors > e1,
      mask DialogControl errorDependentDerivativeOrderDescription3 Prompt: - order = o2 for e2 < error <= e1,
      mask DialogControl errorDependentDerivativeOrderDescription4 Prompt: - order = o3 for e3 < error <= e2,
      mask DialogControl errorDependentDerivativeOrderDescription5 Prompt: - order = o4 for error < e3.
      mask DialogControl timeDependentDerivativeOrderDescription1 Prompt: Insert short expression which returns value of order as a function of time (t) and/or control error (e), e.g.: '2*t + e' (where 't' is current simulation time and 'e' is current value of the control error).
  GL FVOPID - convolution type (external orders) : Subsystem  mask{kp=1, ki=1, kd=0, sampleTime=1, inputBufferSize=-1, constantIntegralOrder=1, constantDerivativeOrder=1, satEnab=off, satHigh=inf, satLow=-inf}
      mask prompts: kp "Proportional (P)"; ki "Integral (I)"; kd "Derivative (D)"; sampleTime "Sample time"; inputBufferSize "Input buffer size (-1 for automatically calculated)"; constantIntegralOrder "Integral order"; constantDerivativeOrder "Derivative order"; satEnab "Limit output"; satHigh "Upper limit"; satLow "Lower limit"
      mask init:
      | % Initialize block parameters
      | fvopidToolbox.library.utils.initializeBasicModelParameters(sampleTime, inputBufferSize,'fvopidConv');
      settings: CopyFcn=set_param(gcbh, 'LinkStatus', 'none');
      mask Callback satEnab:
      | limitOutputCheckBoxValue = get_param(gcb,'satEnab');
      | if strcmp(limitOutputCheckBoxValue, 'on')
      |    fvopidToolbox.library.utils.setMaskParameterPropertyValue('satHigh', 'MaskEnables', 'on');
      |    fvopidToolbox.library.utils.setMaskParameterPropertyValue('satLow', 'MaskEnables', 'on');
      | else
      |    fvopidToolbox.library.utils.setMaskParameterPropertyValue('satHigh', 'MaskEnables', 'off');
      |    fvopidToolbox.library.utils.setMaskParameterPropertyValue('satLow', 'MaskEnables', 'off');
      | end
      mask DialogControl mainTab Prompt: Main
      mask DialogControl controllerParametersGroupBox Prompt: Controller parameters
      mask DialogControl outputSaturationTab Prompt: Output saturation
      mask DialogControl outputSaturationGroupBox Prompt: Output saturation
